simulink model "simulation_version2021b"  (R2021b)
settings: Solver=ode113  StartTime=0.0  StopTime=9  FixedStep=0.001  RelTol=1e-2
values from neighbouring files (symbols this model uses):
  b0 = 0.1    [Parameters.m]
  beta01 = 3000    [Parameters.m]
  beta02 = 100    [Parameters.m]
  beta03 = 0.01    [Parameters.m]
  d = 0.707    [Parameters.m]
  J = 8e-6    (= 8e-06)    [Parameters.m]
  k = 0.2    [Parameters.m]
  L = 0.00525    [Parameters.m]
  lambda_r = 0.0499006    [Parameters.m]
  P = 6    [Parameters.m]
  R = 7.5    [Parameters.m]
libraries: simulink x1
settings Model: Creator=49266  LastModifiedBy=49266
settings SolverCC: ZeroCrossAlgorithm=Adaptive
settings DebuggingCC: MaskedZcDiagnostic=none  IgnoredZcDiagnostic=none

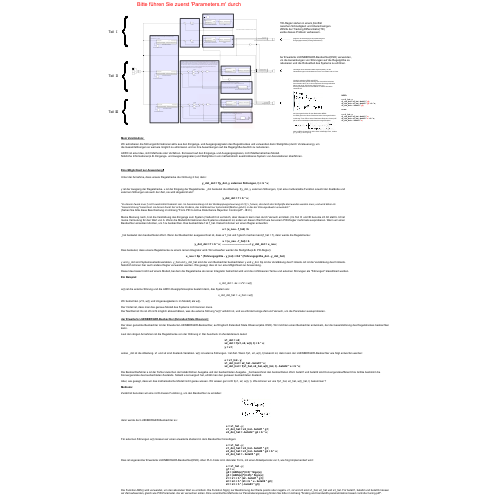
[thumbnail: Simulink's stored preview of the top-level diagram]
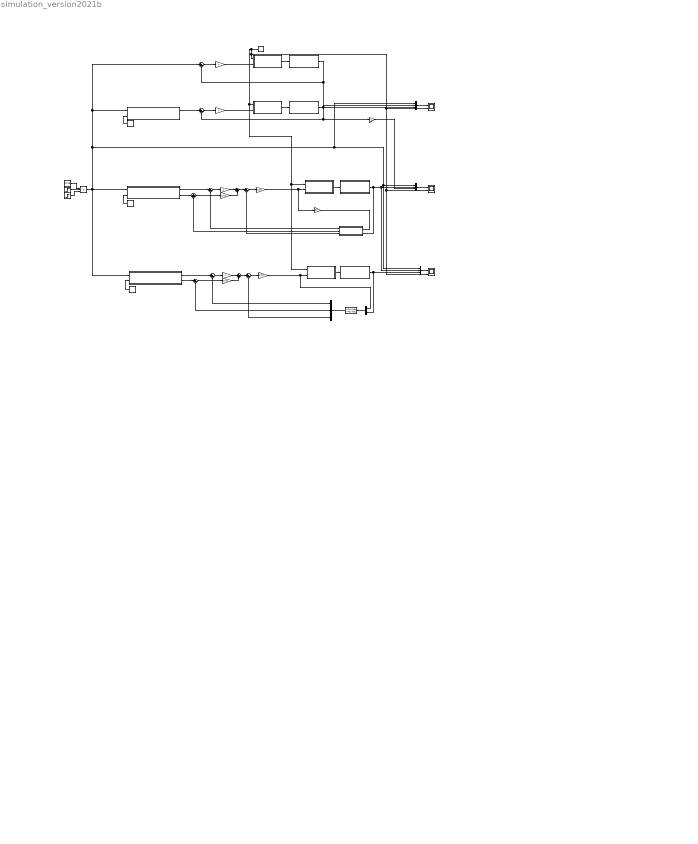
== system simulation_version2021b ==
  note: NESO:
      |
      | e = x1_hat - y;
      | x1_dot_hat = x2_hat - beta01 * g1 ;
      | x2_dot_hat = x3_hat - beta02 * g2 + b * u;
      | x3_dot_hat = - beta03 * g3 ;
  note: der Erweiterte LUENBERGER-Beobachter (Extended State Observer):
      |
      | Der oben genannte Beobachter ist der Erweiterte LUENBERGER-Beobachter, auf Englisch Extended State Observer(abk. ESO). Wir möchten einen Beobachter entwickeln, der die Gesamtstörung des Regelstreckes beobachten kann.
      |
      | Laut den obigen Annahmen ist die Regelstrecke von der Ordnung 2. Der Ausdruck im Zustandsraum lautet:
      |
      | x1_dot = x2;
      | x2_dot = f(x1, x2, w(t), t) + b * u;
      | y = x1;
      |
      | wobei _dot ist die Ableitung. x1 und x2 sind Zustand-Variablen. w(t) ist externe Störungen. t ist Zeit. Wenn f(x1, x2, w(t), t) bekannt ist, dann kann der LUENBERGER-Beobachter wie folgt entworfen werden:
      |
      | e = x1_hat - y;
      | x1_dot_hat = x2_hat - beta01 * e;
      | x2_dot_hat = f(x1_hat, x2_hat, w(t)_hat, t) - beta02 * e + b *u;
      |
      | Die Beobachterfehler e ist der Fehler zwischen der tatsächlichen Ausgabe und der beobachteten Ausgabe. _hat bezeichnet den beobachteten Wert. beta01 und beta02 sind Konvergenzkoeffizient.Ihre Größe bestimmt die Konvergenzrate des beobachteten Zustands. Sobald e konvergiert hat, erhält man den genauen beobachteten Zustand.
      |
      | Aber, wie gesagt, dass wir das mathematische Modell nicht genau wissen. Wir wissen gar nicht f(x1, x2, w(t), t). Wie können wir uns f(x1_hat, x2_hat, w(t)_hat, t) bekommen？
      |
      | Methode:
      |
      | Zunächst benutzen wir eine nicht-lineare Funktion g, um den Beobachter zu erstellen:
      |
      | dann werde der LUENBERGER-Beobachter so:
      |
      | e = x1_hat - y;
      | x1_dot_hat = x2_hat - beta01 * g1;
      | x2_dot_hat = -beta02 * g2 + b * u;
      |
      | Für externen Störungen w(t) müssen wir einen erweiterte Zustand in dem Beobachter hinzufügen:
      |
      | e = x1_hat - y;
      | x1_dot_hat = x2_hat - beta01 * g1;
      | x2_dot_hat = x3_hat - beta02 * g2 + b * u;
      | x3_dot_hat = - beta03 * g3;
      |
      | Dies ist sogenannter Erweiterte LUENBERGER-Beobachter(ESO). Aber PLC-Code ist in diskreter Form, mit einer Abtastperiode von h, wie folgt implementiert wird:
      |
      | e = x1_hat - y;
      | g1 = e;
      | g2 = (ABS(e))^(0.5) * Sign(e);
      | g3 = (ABS(e))^(0.25) * Sign(e);
      | z1 = z1 + h * (z2 - beta01 * g1);
      | z2 = z2 + h * (z3 + b * u - beta02 * g2);
      | z3 = z3 + h * (- beta03 * g3);
      |
      | Die Funktion ABS() wird verwendet, um den absoluten Wert zu ermitteln. Die Funktion Sign() zur Bestimmung der Werte positiv oder negativ. z1, z2 und z3 sind x1_hat, x2_hat und x3_hat. Für beta01, beta02 und beta03 müssen wir Zeit aufwenden, gleich wie PID-Parameter. die wir versuchen sollen. Eine vereinfachte Methode zur Parameteranpassung finden Sie bitte im Anhang "Scaling and bandwidth-parametrization based controller tuning.pdf".
  note: der Erweiterte LUENBERGER-Beobachter(ESO) verwenden, um die Auswirkungen von Störungen auf die Regelgröße zu reduzieren und die Robustheit des Systems zu erhöhen.
  note: PID-Regler stehen in einem Konflikt zwischen Schnelligkeit und Überschwingen.
      | Mithilfe der Tracking Differentiator(TD) werde dieses Problem verbessern.
  note: Regelstrecke
  note: Regelstrecke
  note: Regelstrecke
  note: Regelstrecke
  note: Bitte führen Sie zuerst 'Parameters.m' durch
  note: Eine Möglichkeit zur Anwendung：
      |
      | Unter der Annahme, dass unsere Regelstrecke die Ordnung 2 hat, dann:
      |
      | y_dot_dot = f(y_dot, y, externen Störungen, t) + b * u;
      |
      | y ist der Ausgang der Regelstrecke. u ist der Eingang der Regelstrecke. _dot bedeutet die Ableitung. f(y_dot, y, externen Störungen, t) ist eine multivariable Funktion sowohl der Zustände und externen Störungen als auch der Zeit, sie wird abgekürzt als f：
      |
      | y_dot_dot = f + b * u;
      |
      | "Zu diesem Zweck muss f nicht ausdrücklich bekannt sein. Im Zusammenhang mit der Rückkopplungssteuerung ist F(t) = f etwas, das durch das Stellgröße überwunden werden muss, und wird daher als "Gesamtstörung" bezeichnet. An diesem Punkt hat sich das Problem, das traditionell zur Systemidentifikation gehört, in das der Störungsabwehr verwandelt."
      | (Sehen Sie bitte diese Beschreibung im Anhang "From PID to Active Disturbance Rejection Control.pdf" - Ⅲ.D.)
      |
      | Meine Meinung nach, b ist die Verstärkung des Eingangs zum System.(Vielleicht ist es falsch, aber dieses b kann man durch Versuch ermitteln.) Im Teil Ⅱ und Ⅲ benutze ich b0 statt b. b0 ist meine Vermutung für den Wert von b. Wenn die Modellinformationen des Systems unbekannt ist, sollen wir diesen Wert b0 wie bei einem PID-Regler mehrmals ausprobieren. Wenn wir einen Beobachter einsetzen könnten, um f zu beobachten. Das beobachtete f ist f_hat. Danach können wir einen Regler entwerfen:
      |
      | u = (u_neu - f_hat) / b
      |
      | _hat bedeutet den beobachteten Wert. Wenn der Beobachter ausgezeichnet ist, dass er f_hat und f gleich machen kann(f_hat = f), dann werde die Regelstrecke:
      |
      | u = (u_neu - f_hat) / b
      | y_dot_dot = f + b * u; -------------------------------> y_dot_dot = u_neu;
      |
      | Dies bedeutet, dass unsere Regelstrecke zu einem reinen Integrator wird. Wir entwerfen weriter die Stellgröße(z.B. PD-Regler):
      |
      | u_neu = Kp * (Führungsgröße - y_hat) + Kd * (Führungsgröße_dot - y_dot_hat)
      |
      | y und y_dot sind Systemzustandsvariablen. y_hat und y_dot_hat sind die vom Beobachter beobachteten y und y_dot. Kp ist die Verstärkung des P-Glieds. kd ist die Verstärkung des D-Glieds. Natürlich können hier auch andere Regler verwendet werden. Wie gesagt, dies ist nur eine Möglichkeit zur Anwendung.
      |
      | Diese Idee basiert nicht auf einem Modell, bei dem die Regelstrecke als reiner Integrator betrachtet wird und die nichtlinearen Terme und externen Störungen als "Störungen" klassifiziert werden.
      |
      | Ein Beispiel:
      |
      | x_dot_dot = -kx + x^2 + w(t)
      |
      | w(t) ist die externe Störung und die ADRC-Designphilosophie besteht darin, das System als:
      |
      | x_dot_dot_hat = -x_hat + w(t)
      |
      | Wir betrachten (x^2, w(t) und Ungenauigkeiten k im Modell) als w(t).
      |
      | Der Vorteil ist, dass man das genaue Modell des Systems nicht kennen muss.
      | Der Nachteil ist: Es ist oft nicht möglich abzuschätzen, was die externe Störung "w(t)" wirklich ist, und es erfordert einige Zeit und Versuch, um die Parameter auszuprobieren.
  note: Mein Verständnis:
      |
      | Wir extrahieren die Störungsinformationen aktiv aus den Eingangs- und Ausgangssignalen des Regelstreckes und verwenden dann Stellgröße (durch Vorsteuerung), um die Gesamtstörungen so weit wie möglich zu eliminieren und so ihre Auswirkungen auf die Regelgröße deutlich zu reduzieren.
      |
      | ADRC ist eine Idee, nicht Methode oder Verfahren. Es basiert auf den Eingangs- und Ausgangssignalen, nicht Mathematisches Modell.
      | Nützliche Informationen(z.B. Eingangs- und Ausgangssignalen) und Stellgröße in ein mathematisch ausdrückbares System von Assoziationen überführen.
  note: Teil Ⅰ
  note: nomaler PID-Regler mit Feedback-Kreis
  note: Linear Extended State Observer (LESO)
      | ist der Erweiterte Lineare LUENBERGER-Beobachter
  note: Nicht-linear Extended State Observer (NESO)
      | ist der Erweiterte Nicht-lineare LUENBERGER-Beobachter
  note: Tracking Differentiator(TD) is a Transient Profile Generator.
      | Um den Konflikt zwischen Schnelligkeit und Überschwingen
      | bei PID-Reglern zu lösen.
  note: Nonlinear Feedback Combination is a Nonlinear Weighted Sum(eigentlich ein PD-Regler).
      | Der ESO ist eigentlich eine Erweiterung des Luenberger Observers mit einer erweiterten Zustand.
      | Dieser erweiterter Zustand wird verwendet, um (den unbekannten Term + externen Störungen +
      | den nicht-linearen Term) zu ermitteln. Dies wird in Abschnitt III.D. der Dissertation beschrieben.
      |
      | Wenn der Extended State Observer (ESO) die Unbekannte(z3) sehr genau ermitteln kann,
      | dann wird die Regelstrecke zu einem reinen Integrator.
  note: Teil Ⅱ
  note: Teil Ⅲ
  note: Vergleich: die Auswirkungen der Anwendung des Übergangsprozesses(Tracking Differentiator)
  note: Hinzufügen eines Extended State Observer(ESO), um die Gesamtstörungen und unbekannten Terme zu ermitteln und zu lösen.
  note: Vergleich zwischen LESO und NESO.
      | Sie haben die fast gleiche Wirkung. Der Unterschied zwischen ihnen besteht darin, ob sie eine nichtlineare Konvergenzfunktion haben oder nicht. Wir können viele Formen von Konvergenzfunktionen für ESO wählen. In dieser Simulation verwende ich
      |
      | als Konvergenzfunktion für den Beobachter NESO.
      | Im LESO gibt es bei dieser Simulation keine Konvergenzfunktion.
      |
      | im Anhang "From PID to Active Disturbance Rejection Control.pdf" gibt es eine vollständige nichtlineare Konvergenzfunktion.
      |
      | Aber in NESO verwende ich nicht diese vollständige Form, sondern g1, g2 und g3. Es ist genug.
  note: LESO:
      |
      | e = x1_hat - y;
      | x1_dot_hat = x2_hat - beta01 * e ;
      | x2_dot_hat = x3_hat - beta02 * e + b * u;
      | x3_dot_hat = - beta03 * e ;
  1/b0 : Gain  Gain=1/b0
  1/b0_1 : Gain  Gain=1/b0
  Aktor(Fadenzugmotor)3 : Subsystem
  Aktor(Servoverstäker+Fadenzugmotor) : Subsystem
  Aktor(Servoverstäker+Fadenzugmotor)1 : Subsystem
  Aktor(Servoverstäker+Fadenzugmotor)2 : Subsystem
  D-Glied : Gain  Gain=0.01
  D-Glied1 : Gain  Gain=0.01
  Demux : Demux  Outputs=3
  Externe Störungen(Einheit: Nm) Motor Rated Torque Mn = 0.38N : simulink/Sources/Band-Limited White Noise  Cov=[0.002]  Ts=0.1  seed=[23341]
  Faden : Subsystem
  Faden1 : Subsystem
  Faden2 : Subsystem
  Faden3 : Subsystem
  Führungsgröße : Product  Inputs=3
  Konvergenzgeschwindigkeit : Constant  Value=2000
  Konvergenzgeschwindigkeit1 : Constant  Value=2000
  Konvergenzgeschwindigkeit2 : Constant  Value=2000
  Linear Extended State Observer (LESO) : StateSpace  A=[-beta01 1 0;-beta02 0 1;-beta03 0 0]  B=[0 beta01;b0 beta02;0 beta03]  C=[1 0 0;0 1 0;0 0 1]  D=[0 0;0 0;0 0]  InitialCondition=0
  Mux : Mux  Inputs=2
  Mux1 : Mux  Inputs=3
  Mux2 : Mux  Inputs=3
  Mux3 : Mux  Inputs=3
  Nicht-linear Extended State Observer (NESO) : Subsystem
  P-Glied{,1..3} (4 alike) : Gain
  Pulse Generator : DiscretePulseGenerator  PulseType=Time based  Amplitude=10  Period=5  PulseWidth=50
  Scope : Scope  NumInputPorts=2
  Scope1 : Scope  NumInputPorts=2
  Scope4 : Scope  NumInputPorts=2
  Step1 : Step  Time=5  Before=1  After=0.5  SampleTime=0
  Step2 : Step  Time=10  Before=1  After=1.5  SampleTime=0
  Sum{,1..3,5,7,9..10} (8 alike) : Sum  Inputs=|+-
  Sum4 : Sum  Inputs=|++
  Sum6 : Sum  Inputs=|++
  Tracking Differentiator(TD) : Subsystem
  Tracking Differentiator(TD)1 : Subsystem
  Tracking Differentiator(TD)2 : Subsystem
  "Um Signal zu umbenennen " : Gain
  b0 : Gain  Gain=b0
  wires:
  Externe Störungen(Einheit: Nm) Motor Rated Torque Mn = 0.38N/1 -> Aktor(Servoverstäker+Fadenzugmotor)1/1(externen Störungen), Aktor(Fadenzugmotor)3/1(externen Störungen), Aktor(Servoverstäker+Fadenzugmotor)2/1(externen Störungen), Scope4/2, Scope1/2, Scope/2, Aktor(Servoverstäker+Fadenzugmotor)/1(externen Störungen)  "Externe Störungen(Einheit: N.m) Motor Rated Torque Mn = 0.38Nm"
  Faden3/1(Fadenzugspannung) -> Mux/2, Mux3/3  "Regelgröße mit LESO"
  Aktor(Fadenzugmotor)3/1(Position) -> Faden3/1(Verdrängung)
  Linear Extended State Observer (LESO)/1 -> Demux/1
  Mux/1 -> Linear Extended State Observer (LESO)/1
  Führungsgröße/1 -> Sum/1, Tracking Differentiator(TD)2/1(Führungsgröße), Mux1/1, Mux3/1, Mux2/1, Tracking Differentiator(TD)/1(Führungsgröße), Tracking Differentiator(TD)1/1(Führungsgröße)  "Führungsgröße"
  P-Glied/1 -> Aktor(Servoverstäker+Fadenzugmotor)/2(Fadenzugspannung)
  Tracking Differentiator(TD)2/1(Übergangskurve) -> Sum1/1
  Step2/1 -> Führungsgröße/3
  Faden2/1(Fadenzugspannung) -> Sum1/2, "Um Signal zu umbenennen "/1, Mux1/3  "mit Tracking Differentiator"
  Sum/1 -> P-Glied/1
  Konvergenzgeschwindigkeit/1 -> Tracking Differentiator(TD)2/2(Konvergenzgeschwindigkeit)
  Pulse Generator/1 -> Führungsgröße/1
  Sum1/1 -> P-Glied1/1
  Step1/1 -> Führungsgröße/2
  P-Glied1/1 -> Aktor(Servoverstäker+Fadenzugmotor)2/2(Fadenzugspannung)
  Faden/1(Fadenzugspannung) -> Mux1/2, Sum/2  "ohne Tracking Differentiator"
  Aktor(Servoverstäker+Fadenzugmotor)/1(Position) -> Faden/1(Verdrängung)
  Aktor(Servoverstäker+Fadenzugmotor)2/1(Position) -> Faden2/1(Verdrängung)
  Aktor(Servoverstäker+Fadenzugmotor)1/1(Position) -> Faden1/1(Verdrängung)
  Faden1/1(Fadenzugspannung) -> Mux3/2, Mux2/2, Nicht-linear Extended State Observer (NESO)/2(y)  "Regelgröße mit ESO"
  Tracking Differentiator(TD)/1(Übergangskurve) -> Sum2/1
  Sum2/1 -> P-Glied3/1
  Konvergenzgeschwindigkeit1/1 -> Tracking Differentiator(TD)/2(Konvergenzgeschwindigkeit)
  Nicht-linear Extended State Observer (NESO)/1(Z1) -> Sum2/2  "x1_hat"
  P-Glied3/1 -> Sum4/1
  Sum4/1 -> Sum9/1
  Tracking Differentiator(TD)/2(Ableitungen der Übergangskurven) -> Sum10/1
  Nicht-linear Extended State Observer (NESO)/2(Z2) -> Sum10/2  "x2_hat"
  Sum10/1 -> D-Glied/1
  Nicht-linear Extended State Observer (NESO)/3(Z3) -> Sum9/2  "x3_hat：total disturbance (Beobachtete Gesamtstörung)"
  Sum9/1 -> 1/b0/1
  1/b0/1 -> b0/1, Aktor(Servoverstäker+Fadenzugmotor)1/2(Fadenzugspannung)
  b0/1 -> Nicht-linear Extended State Observer (NESO)/1(u)
  Demux/3 -> Sum7/2  "x3_hat：total disturbance (Beobachtete Gesamtstörung)"
  Demux/1 -> Sum5/2  "x1_hat"
  Demux/2 -> Sum3/2  "x2_hat"
  D-Glied1/1 -> Sum6/2
  Sum7/1 -> 1/b0_1/1
  1/b0_1/1 -> Mux/1, Aktor(Fadenzugmotor)3/2(Fadenzugspannung)
  Sum3/1 -> D-Glied1/1
  Sum6/1 -> Sum7/1
  P-Glied2/1 -> Sum6/1
  Sum5/1 -> P-Glied2/1
  Konvergenzgeschwindigkeit2/1 -> Tracking Differentiator(TD)1/2(Konvergenzgeschwindigkeit)
  Tracking Differentiator(TD)1/1(Übergangskurve) -> Sum5/1
  Tracking Differentiator(TD)1/2(Ableitungen der Übergangskurven) -> Sum3/1
  "Um Signal zu umbenennen "/1 -> Mux2/3  "Regelgröße ohne ESO"
  Mux1/1 -> Scope/1
  Mux2/1 -> Scope4/1
  Mux3/1 -> Scope1/1
  D-Glied/1 -> Sum4/2

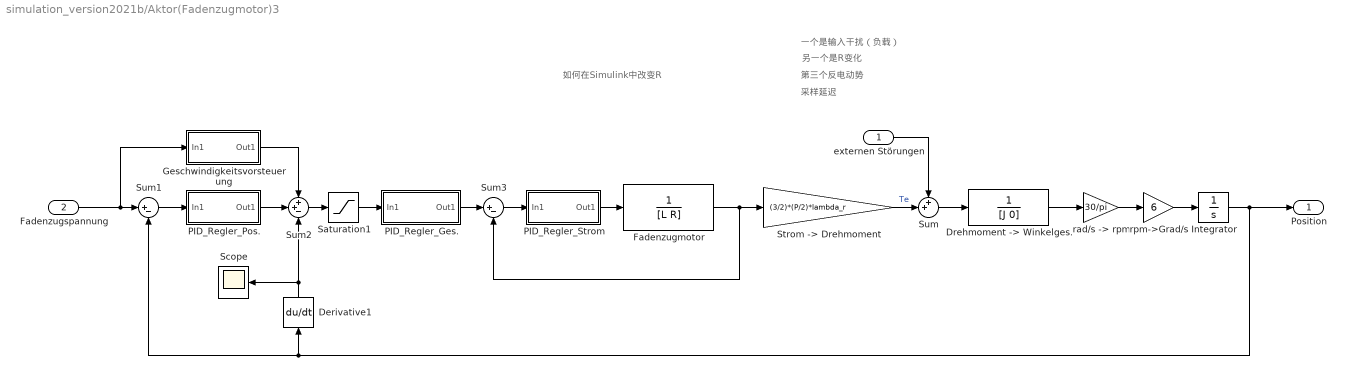
== system simulation_version2021b/Aktor(Fadenzugmotor)3 ==
  note: 采样延迟
  note: 第三个反电动势
  note: 另一个是R变化
  note: 一个是输入干扰（负载）
  note: 如何在Simulink中改变R
  externen Störungen : Inport
  Fadenzugspannung : Inport  Port=2
  Derivative1 : Derivative
  "Drehmoment -> Winkelges." : TransferFcn  Denominator=[J 0]
  Fadenzugmotor : TransferFcn  Denominator=[L R]
  Geschwindigkeitsvorsteuerung : Subsystem
  Integrator : Integrator
  PID_Regler_Ges. : Subsystem
  PID_Regler_Pos. : Subsystem
  PID_Regler_Strom : Subsystem
  Saturation1 : Saturate  UpperLimit=9500  LowerLimit=-9500
  Scope : Scope
  "Strom -> Drehmoment" : Gain  Gain=(3/2)*(P/2)*lambda_r
  Sum : Sum  Inputs=++|
  Sum1 : Sum  Inputs=|+-
  Sum2 : Sum  Inputs=++-
  Sum3 : Sum  Inputs=|+-
  "rad/s -> rpm" : Gain  Gain=30/pi
  rpm->Grad/s : Gain  Gain=6
  Position : Outport
  wires:
  "Drehmoment -> Winkelges."/1 -> "rad/s -> rpm"/1
  Derivative1/1 -> Sum2/3, Scope/1
  Fadenzugspannung/1 -> Geschwindigkeitsvorsteuerung/1(In1), Sum1/1
  rpm->Grad/s/1 -> Integrator/1
  "rad/s -> rpm"/1 -> rpm->Grad/s/1
  Integrator/1 -> Position/1, Derivative1/1, Sum1/2
  Fadenzugmotor/1 -> "Strom -> Drehmoment"/1, Sum3/2
  "Strom -> Drehmoment"/1 -> Sum/2  "Te"
  Sum/1 -> "Drehmoment -> Winkelges."/1
  externen Störungen/1 -> Sum/1
  Sum2/1 -> Saturation1/1
  Saturation1/1 -> PID_Regler_Ges./1(In1)
  PID_Regler_Ges./1(Out1) -> Sum3/1
  Sum1/1 -> PID_Regler_Pos./1(In1)
  PID_Regler_Pos./1(Out1) -> Sum2/2
  Geschwindigkeitsvorsteuerung/1(Out1) -> Sum2/1
  Sum3/1 -> PID_Regler_Strom/1(In1)
  PID_Regler_Strom/1(Out1) -> Fadenzugmotor/1

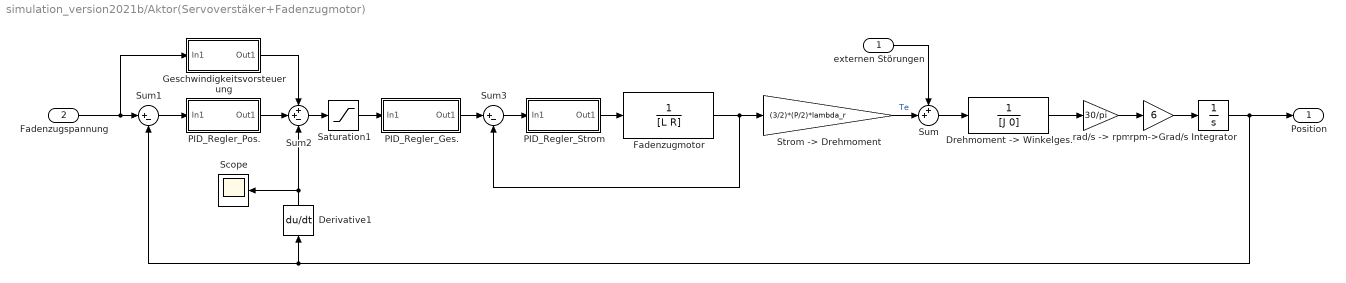
== system simulation_version2021b/Aktor(Servoverstäker+Fadenzugmotor) ==
  externen Störungen : Inport
  Fadenzugspannung : Inport  Port=2
  Derivative1 : Derivative
  "Drehmoment -> Winkelges." : TransferFcn  Denominator=[J 0]
  Fadenzugmotor : TransferFcn  Denominator=[L R]
  Geschwindigkeitsvorsteuerung : Subsystem
  Integrator : Integrator
  PID_Regler_Ges. : Subsystem
  PID_Regler_Pos. : Subsystem
  PID_Regler_Strom : Subsystem
  Saturation1 : Saturate  UpperLimit=9500  LowerLimit=-9500
  Scope : Scope
  "Strom -> Drehmoment" : Gain  Gain=(3/2)*(P/2)*lambda_r
  Sum : Sum  Inputs=++|
  Sum1 : Sum  Inputs=|+-
  Sum2 : Sum  Inputs=++-
  Sum3 : Sum  Inputs=|+-
  "rad/s -> rpm" : Gain  Gain=30/pi
  rpm->Grad/s : Gain  Gain=6
  Position : Outport
  wires:
  "Drehmoment -> Winkelges."/1 -> "rad/s -> rpm"/1
  Derivative1/1 -> Sum2/3, Scope/1
  Fadenzugspannung/1 -> Geschwindigkeitsvorsteuerung/1(In1), Sum1/1
  rpm->Grad/s/1 -> Integrator/1
  "rad/s -> rpm"/1 -> rpm->Grad/s/1
  Integrator/1 -> Position/1, Derivative1/1, Sum1/2
  Fadenzugmotor/1 -> "Strom -> Drehmoment"/1, Sum3/2
  "Strom -> Drehmoment"/1 -> Sum/2  "Te"
  Sum/1 -> "Drehmoment -> Winkelges."/1
  externen Störungen/1 -> Sum/1
  Sum2/1 -> Saturation1/1
  Saturation1/1 -> PID_Regler_Ges./1(In1)
  PID_Regler_Ges./1(Out1) -> Sum3/1
  Sum1/1 -> PID_Regler_Pos./1(In1)
  PID_Regler_Pos./1(Out1) -> Sum2/2
  Geschwindigkeitsvorsteuerung/1(Out1) -> Sum2/1
  Sum3/1 -> PID_Regler_Strom/1(In1)
  PID_Regler_Strom/1(Out1) -> Fadenzugmotor/1

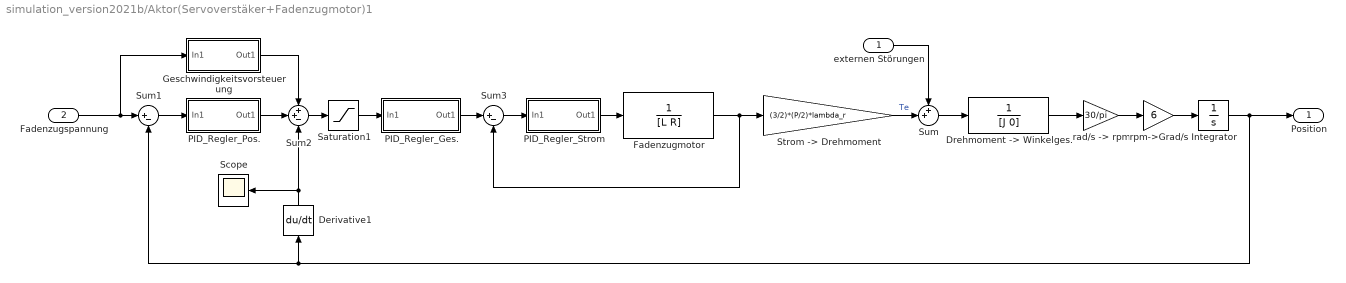
== system simulation_version2021b/Aktor(Servoverstäker+Fadenzugmotor)1 ==
  externen Störungen : Inport
  Fadenzugspannung : Inport  Port=2
  Derivative1 : Derivative
  "Drehmoment -> Winkelges." : TransferFcn  Denominator=[J 0]
  Fadenzugmotor : TransferFcn  Denominator=[L R]
  Geschwindigkeitsvorsteuerung : Subsystem
  Integrator : Integrator
  PID_Regler_Ges. : Subsystem
  PID_Regler_Pos. : Subsystem
  PID_Regler_Strom : Subsystem
  Saturation1 : Saturate  UpperLimit=9500  LowerLimit=-9500
  Scope : Scope
  "Strom -> Drehmoment" : Gain  Gain=(3/2)*(P/2)*lambda_r
  Sum : Sum  Inputs=++|
  Sum1 : Sum  Inputs=|+-
  Sum2 : Sum  Inputs=++-
  Sum3 : Sum  Inputs=|+-
  "rad/s -> rpm" : Gain  Gain=30/pi
  rpm->Grad/s : Gain  Gain=6
  Position : Outport
  wires:
  "Drehmoment -> Winkelges."/1 -> "rad/s -> rpm"/1
  Derivative1/1 -> Sum2/3, Scope/1
  Fadenzugspannung/1 -> Geschwindigkeitsvorsteuerung/1(In1), Sum1/1
  rpm->Grad/s/1 -> Integrator/1
  "rad/s -> rpm"/1 -> rpm->Grad/s/1
  Integrator/1 -> Position/1, Derivative1/1, Sum1/2
  Fadenzugmotor/1 -> "Strom -> Drehmoment"/1, Sum3/2
  "Strom -> Drehmoment"/1 -> Sum/2  "Te"
  Sum/1 -> "Drehmoment -> Winkelges."/1
  externen Störungen/1 -> Sum/1
  Sum2/1 -> Saturation1/1
  Saturation1/1 -> PID_Regler_Ges./1(In1)
  PID_Regler_Ges./1(Out1) -> Sum3/1
  Sum1/1 -> PID_Regler_Pos./1(In1)
  PID_Regler_Pos./1(Out1) -> Sum2/2
  Geschwindigkeitsvorsteuerung/1(Out1) -> Sum2/1
  Sum3/1 -> PID_Regler_Strom/1(In1)
  PID_Regler_Strom/1(Out1) -> Fadenzugmotor/1

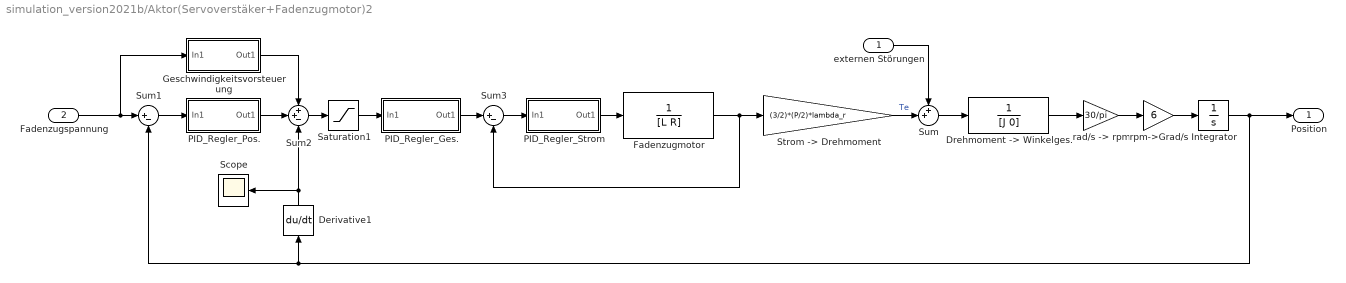
== system simulation_version2021b/Aktor(Servoverstäker+Fadenzugmotor)2 ==
  externen Störungen : Inport
  Fadenzugspannung : Inport  Port=2
  Derivative1 : Derivative
  "Drehmoment -> Winkelges." : TransferFcn  Denominator=[J 0]
  Fadenzugmotor : TransferFcn  Denominator=[L R]
  Geschwindigkeitsvorsteuerung : Subsystem
  Integrator : Integrator
  PID_Regler_Ges. : Subsystem
  PID_Regler_Pos. : Subsystem
  PID_Regler_Strom : Subsystem
  Saturation1 : Saturate  UpperLimit=9500  LowerLimit=-9500
  Scope : Scope
  "Strom -> Drehmoment" : Gain  Gain=(3/2)*(P/2)*lambda_r
  Sum : Sum  Inputs=++|
  Sum1 : Sum  Inputs=|+-
  Sum2 : Sum  Inputs=++-
  Sum3 : Sum  Inputs=|+-
  "rad/s -> rpm" : Gain  Gain=30/pi
  rpm->Grad/s : Gain  Gain=6
  Position : Outport
  wires:
  "Drehmoment -> Winkelges."/1 -> "rad/s -> rpm"/1
  Derivative1/1 -> Sum2/3, Scope/1
  Fadenzugspannung/1 -> Geschwindigkeitsvorsteuerung/1(In1), Sum1/1
  rpm->Grad/s/1 -> Integrator/1
  "rad/s -> rpm"/1 -> rpm->Grad/s/1
  Integrator/1 -> Position/1, Derivative1/1, Sum1/2
  Fadenzugmotor/1 -> "Strom -> Drehmoment"/1, Sum3/2
  "Strom -> Drehmoment"/1 -> Sum/2  "Te"
  Sum/1 -> "Drehmoment -> Winkelges."/1
  externen Störungen/1 -> Sum/1
  Sum2/1 -> Saturation1/1
  Saturation1/1 -> PID_Regler_Ges./1(In1)
  PID_Regler_Ges./1(Out1) -> Sum3/1
  Sum1/1 -> PID_Regler_Pos./1(In1)
  PID_Regler_Pos./1(Out1) -> Sum2/2
  Geschwindigkeitsvorsteuerung/1(Out1) -> Sum2/1
  Sum3/1 -> PID_Regler_Strom/1(In1)
  PID_Regler_Strom/1(Out1) -> Fadenzugmotor/1

== system simulation_version2021b/Faden ==
  Verdrängung : Inport
  Transfer Fcn : TransferFcn  Numerator=[400]  Denominator=[d k]
  Fadenzugspannung : Outport
  wires:
  Verdrängung/1 -> Transfer Fcn/1
  Transfer Fcn/1 -> Fadenzugspannung/1

== system simulation_version2021b/Faden1 ==
  Verdrängung : Inport
  Transfer Fcn : TransferFcn  Numerator=[400]  Denominator=[d k]
  Fadenzugspannung : Outport
  wires:
  Verdrängung/1 -> Transfer Fcn/1
  Transfer Fcn/1 -> Fadenzugspannung/1

== system simulation_version2021b/Faden2 ==
  Verdrängung : Inport
  Transfer Fcn : TransferFcn  Numerator=[400]  Denominator=[d k]
  Fadenzugspannung : Outport
  wires:
  Transfer Fcn/1 -> Fadenzugspannung/1
  Verdrängung/1 -> Transfer Fcn/1

== system simulation_version2021b/Faden3 ==
  Verdrängung : Inport
  Transfer Fcn : TransferFcn  Numerator=[400]  Denominator=[d k]
  Fadenzugspannung : Outport
  wires:
  Transfer Fcn/1 -> Fadenzugspannung/1
  Verdrängung/1 -> Transfer Fcn/1

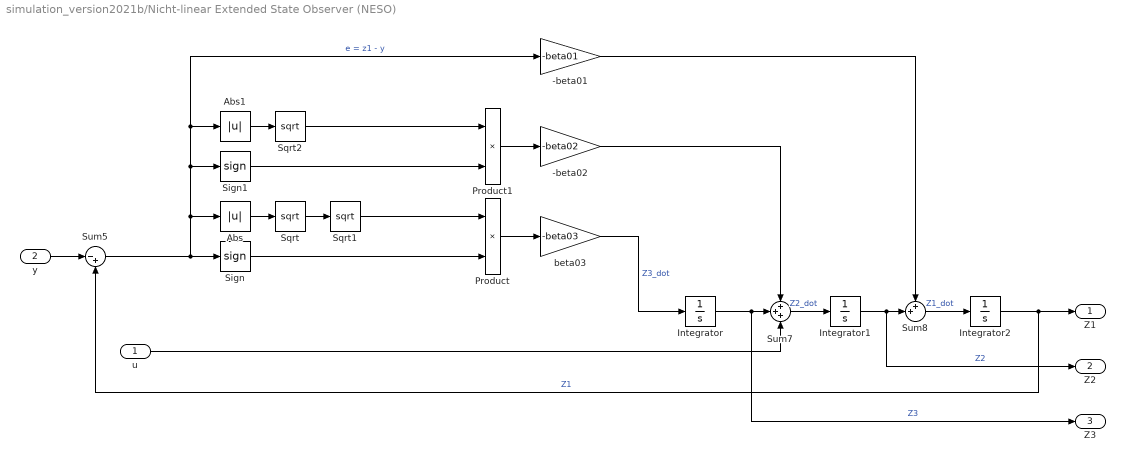
== system simulation_version2021b/Nicht-linear Extended State Observer (NESO) ==
  u : Inport
  y : Inport  Port=2
  -beta01 : Gain  Gain=-beta01
  -beta02 : Gain  Gain=-beta02
  Abs : Abs
  Abs1 : Abs
  Integrator : Integrator
  Integrator1 : Integrator
  Integrator2 : Integrator
  Product : Product
  Product1 : Product
  Sign : Signum
  Sign1 : Signum
  Sqrt : Sqrt  SaturateOnIntegerOverflow=on
  Sqrt1 : Sqrt  SaturateOnIntegerOverflow=on
  Sqrt2 : Sqrt  SaturateOnIntegerOverflow=on
  Sum5 : Sum  Inputs=|-+
  Sum7 : Sum  Inputs=+++
  Sum8 : Sum  Inputs=++|
  beta03 : Gain  Gain=-beta03
  Z1 : Outport
  Z2 : Outport  Port=2
  Z3 : Outport  Port=3
  wires:
  Abs/1 -> Sqrt/1
  Sqrt/1 -> Sqrt1/1
  beta03/1 -> Integrator/1  "Z3_dot"
  Integrator1/1 -> Sum8/2, Z2/1  "Z2"
  Sum5/1 -> Sign1/1, -beta01/1, Abs1/1, Abs/1, Sign/1  "e = z1 - y"
  Integrator2/1 -> Z1/1, Sum5/2  "Z1"
  Sign1/1 -> Product1/2
  Abs1/1 -> Sqrt2/1
  Sum8/1 -> Integrator2/1  "Z1_dot"
  Sum7/1 -> Integrator1/1  "Z2_dot"
  Product1/1 -> -beta02/1
  -beta02/1 -> Sum7/1
  Product/1 -> beta03/1
  -beta01/1 -> Sum8/1
  Sign/1 -> Product/2
  Integrator/1 -> Z3/1, Sum7/2  "Z3"
  y/1 -> Sum5/1
  Sqrt1/1 -> Product/1
  u/1 -> Sum7/3
  Sqrt2/1 -> Product1/1

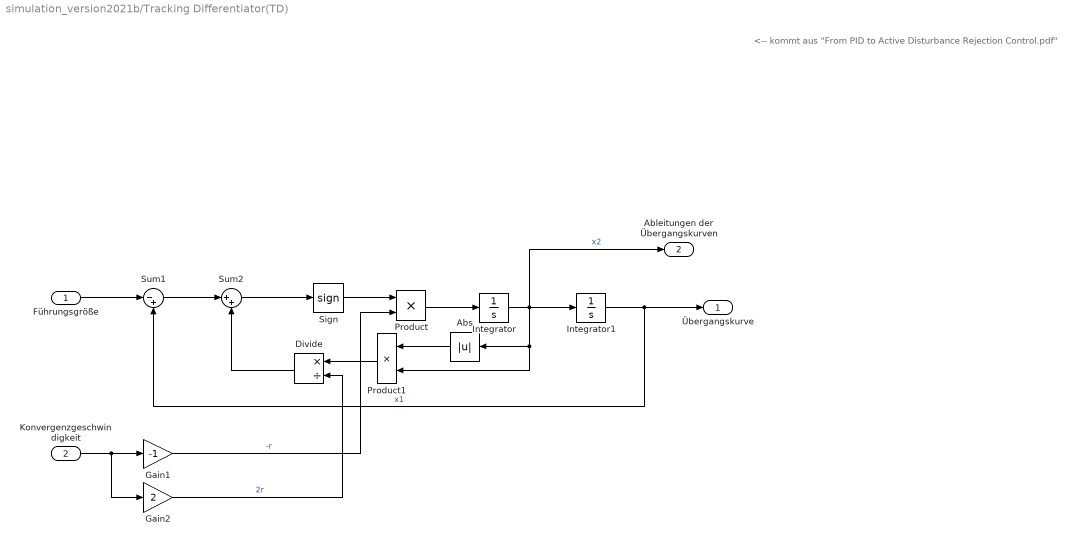
== system simulation_version2021b/Tracking Differentiator(TD) ==
  note: <-- kommt aus "From PID to Active Disturbance Rejection Control.pdf"
  Führungsgröße : Inport
  Konvergenzgeschwindigkeit : Inport  Port=2
  Abs : Abs
  Divide : Product  Inputs=*/
  Gain1 : Gain  Gain=-1
  Gain2 : Gain  Gain=2
  Integrator : Integrator
  Integrator1 : Integrator
  Product : Product
  Product1 : Product
  Sign : Signum
  Sum1 : Sum  Inputs=|-+
  Sum2 : Sum  Inputs=|++
  Übergangskurve : Outport
  Ableitungen der Übergangskurven : Outport  Port=2
  wires:
  Sum1/1 -> Sum2/1
  Product1/1 -> Divide/1
  Konvergenzgeschwindigkeit/1 -> Gain2/1, Gain1/1
  Führungsgröße/1 -> Sum1/1
  Integrator/1 -> Ableitungen der Übergangskurven/1, Integrator1/1, Product1/2, Abs/1  "x2"
  Divide/1 -> Sum2/2
  Integrator1/1 -> Übergangskurve/1, Sum1/2  "x1"
  Product/1 -> Integrator/1
  Abs/1 -> Product1/1
  Sum2/1 -> Sign/1
  Gain1/1 -> Product/2  "-r"
  Sign/1 -> Product/1
  Gain2/1 -> Divide/2  "2r"

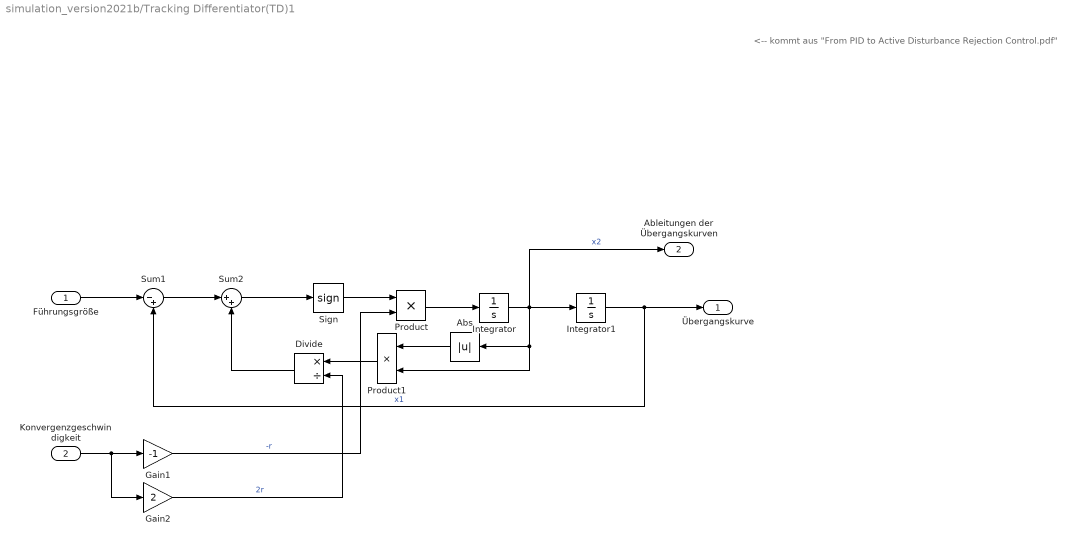
== system simulation_version2021b/Tracking Differentiator(TD)1 ==
  note: <-- kommt aus "From PID to Active Disturbance Rejection Control.pdf"
  Führungsgröße : Inport
  Konvergenzgeschwindigkeit : Inport  Port=2
  Abs : Abs
  Divide : Product  Inputs=*/
  Gain1 : Gain  Gain=-1
  Gain2 : Gain  Gain=2
  Integrator : Integrator
  Integrator1 : Integrator
  Product : Product
  Product1 : Product
  Sign : Signum
  Sum1 : Sum  Inputs=|-+
  Sum2 : Sum  Inputs=|++
  Übergangskurve : Outport
  Ableitungen der Übergangskurven : Outport  Port=2
  wires:
  Sum1/1 -> Sum2/1
  Product1/1 -> Divide/1
  Konvergenzgeschwindigkeit/1 -> Gain2/1, Gain1/1
  Führungsgröße/1 -> Sum1/1
  Integrator/1 -> Ableitungen der Übergangskurven/1, Integrator1/1, Product1/2, Abs/1  "x2"
  Divide/1 -> Sum2/2
  Integrator1/1 -> Übergangskurve/1, Sum1/2  "x1"
  Product/1 -> Integrator/1
  Abs/1 -> Product1/1
  Sum2/1 -> Sign/1
  Gain1/1 -> Product/2  "-r"
  Sign/1 -> Product/1
  Gain2/1 -> Divide/2  "2r"

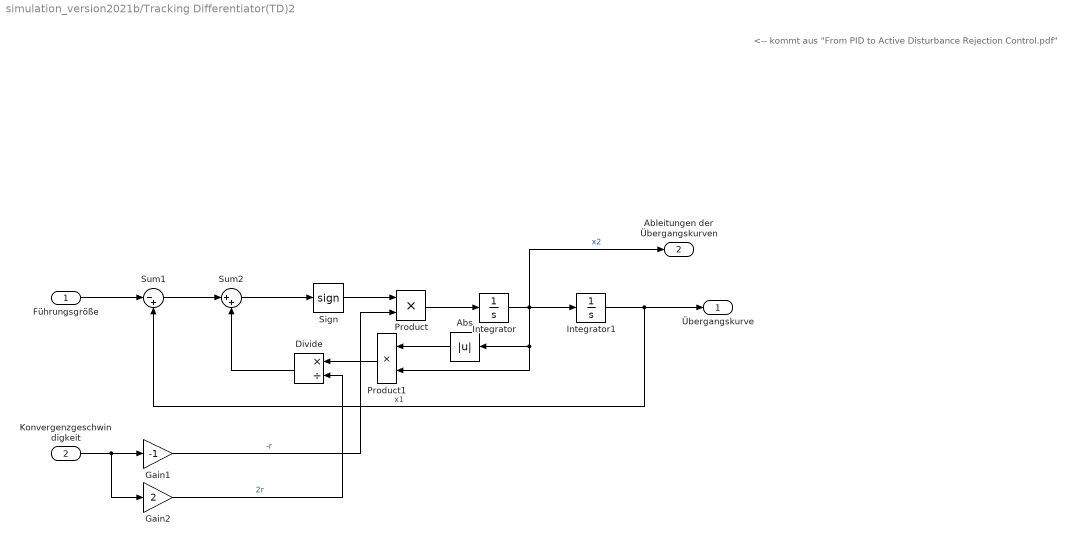
== system simulation_version2021b/Tracking Differentiator(TD)2 ==
  note: <-- kommt aus "From PID to Active Disturbance Rejection Control.pdf"
  Führungsgröße : Inport
  Konvergenzgeschwindigkeit : Inport  Port=2
  Abs : Abs
  Divide : Product  Inputs=*/
  Gain1 : Gain  Gain=-1
  Gain2 : Gain  Gain=2
  Integrator : Integrator
  Integrator1 : Integrator
  Product : Product
  Product1 : Product
  Sign : Signum
  Sum1 : Sum  Inputs=|-+
  Sum2 : Sum  Inputs=|++
  Übergangskurve : Outport
  Ableitungen der Übergangskurven : Outport  Port=2
  wires:
  Gain2/1 -> Divide/2  "2r"
  Sign/1 -> Product/1
  Gain1/1 -> Product/2  "-r"
  Sum2/1 -> Sign/1
  Abs/1 -> Product1/1
  Product/1 -> Integrator/1
  Integrator1/1 -> Sum1/2, Übergangskurve/1  "x1"
  Divide/1 -> Sum2/2
  Integrator/1 -> Abs/1, Product1/2, Integrator1/1, Ableitungen der Übergangskurven/1  "x2"
  Führungsgröße/1 -> Sum1/1
  Konvergenzgeschwindigkeit/1 -> Gain1/1, Gain2/1
  Product1/1 -> Divide/1
  Sum1/1 -> Sum2/1

== system simulation_version2021b/Aktor(Fadenzugmotor)3/Geschwindigkeitsvorsteuerung ==
  In1 : Inport
  Derivative : Derivative
  Gain : Gain
  Out1 : Outport
  wires:
  Derivative/1 -> Gain/1
  In1/1 -> Derivative/1
  Gain/1 -> Out1/1

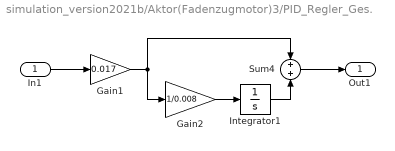
== system simulation_version2021b/Aktor(Fadenzugmotor)3/PID_Regler_Ges. ==
  In1 : Inport
  Gain1 : Gain  Gain=0.017
  Gain2 : Gain  Gain=1/0.008
  Integrator1 : Integrator
  Sum4 : Sum  Inputs=+|+
  Out1 : Outport
  wires:
  Integrator1/1 -> Sum4/2
  Gain1/1 -> Gain2/1, Sum4/1
  Gain2/1 -> Integrator1/1
  Sum4/1 -> Out1/1
  In1/1 -> Gain1/1

== system simulation_version2021b/Aktor(Fadenzugmotor)3/PID_Regler_Pos. ==
  In1 : Inport
  Gain3 : Gain  Gain=4
  Out1 : Outport
  wires:
  Gain3/1 -> Out1/1
  In1/1 -> Gain3/1

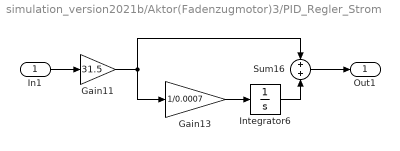
== system simulation_version2021b/Aktor(Fadenzugmotor)3/PID_Regler_Strom ==
  In1 : Inport
  Gain11 : Gain  Gain=31.5
  Gain13 : Gain  Gain=1/0.0007
  Integrator6 : Integrator
  Sum16 : Sum  Inputs=+|+
  Out1 : Outport
  wires:
  Gain13/1 -> Integrator6/1
  Gain11/1 -> Gain13/1, Sum16/1
  In1/1 -> Gain11/1
  Sum16/1 -> Out1/1
  Integrator6/1 -> Sum16/2

== system simulation_version2021b/Aktor(Servoverstäker+Fadenzugmotor)/Geschwindigkeitsvorsteuerung ==
  In1 : Inport
  Derivative : Derivative
  Gain : Gain
  Out1 : Outport
  wires:
  Derivative/1 -> Gain/1
  In1/1 -> Derivative/1
  Gain/1 -> Out1/1

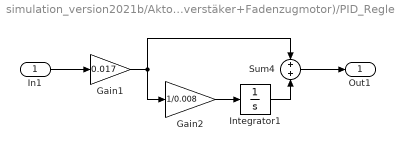
== system simulation_version2021b/Aktor(Servoverstäker+Fadenzugmotor)/PID_Regler_Ges. ==
  In1 : Inport
  Gain1 : Gain  Gain=0.017
  Gain2 : Gain  Gain=1/0.008
  Integrator1 : Integrator
  Sum4 : Sum  Inputs=+|+
  Out1 : Outport
  wires:
  Integrator1/1 -> Sum4/2
  Gain1/1 -> Gain2/1, Sum4/1
  Gain2/1 -> Integrator1/1
  Sum4/1 -> Out1/1
  In1/1 -> Gain1/1

== system simulation_version2021b/Aktor(Servoverstäker+Fadenzugmotor)/PID_Regler_Pos. ==
  In1 : Inport
  Gain3 : Gain  Gain=4
  Out1 : Outport
  wires:
  Gain3/1 -> Out1/1
  In1/1 -> Gain3/1

== system simulation_version2021b/Aktor(Servoverstäker+Fadenzugmotor)/PID_Regler_Strom ==
  In1 : Inport
  Gain11 : Gain  Gain=31.5
  Gain13 : Gain  Gain=1/0.0007
  Integrator6 : Integrator
  Sum16 : Sum  Inputs=+|+
  Out1 : Outport
  wires:
  Gain13/1 -> Integrator6/1
  Gain11/1 -> Gain13/1, Sum16/1
  In1/1 -> Gain11/1
  Sum16/1 -> Out1/1
  Integrator6/1 -> Sum16/2

== system simulation_version2021b/Aktor(Servoverstäker+Fadenzugmotor)1/Geschwindigkeitsvorsteuerung ==
  In1 : Inport
  Derivative : Derivative
  Gain : Gain
  Out1 : Outport
  wires:
  Derivative/1 -> Gain/1
  In1/1 -> Derivative/1
  Gain/1 -> Out1/1

== system simulation_version2021b/Aktor(Servoverstäker+Fadenzugmotor)1/PID_Regler_Ges. ==
  In1 : Inport
  Gain1 : Gain  Gain=0.017
  Gain2 : Gain  Gain=1/0.008
  Integrator1 : Integrator
  Sum4 : Sum  Inputs=+|+
  Out1 : Outport
  wires:
  Integrator1/1 -> Sum4/2
  Gain1/1 -> Gain2/1, Sum4/1
  Gain2/1 -> Integrator1/1
  Sum4/1 -> Out1/1
  In1/1 -> Gain1/1

== system simulation_version2021b/Aktor(Servoverstäker+Fadenzugmotor)1/PID_Regler_Pos. ==
  In1 : Inport
  Gain3 : Gain  Gain=4
  Out1 : Outport
  wires:
  Gain3/1 -> Out1/1
  In1/1 -> Gain3/1

== system simulation_version2021b/Aktor(Servoverstäker+Fadenzugmotor)1/PID_Regler_Strom ==
  In1 : Inport
  Gain11 : Gain  Gain=31.5
  Gain13 : Gain  Gain=1/0.0007
  Integrator6 : Integrator
  Sum16 : Sum  Inputs=+|+
  Out1 : Outport
  wires:
  Gain13/1 -> Integrator6/1
  Gain11/1 -> Gain13/1, Sum16/1
  In1/1 -> Gain11/1
  Sum16/1 -> Out1/1
  Integrator6/1 -> Sum16/2

== system simulation_version2021b/Aktor(Servoverstäker+Fadenzugmotor)2/Geschwindigkeitsvorsteuerung ==
  In1 : Inport
  Derivative : Derivative
  Gain : Gain
  Out1 : Outport
  wires:
  Derivative/1 -> Gain/1
  In1/1 -> Derivative/1
  Gain/1 -> Out1/1

== system simulation_version2021b/Aktor(Servoverstäker+Fadenzugmotor)2/PID_Regler_Ges. ==
  In1 : Inport
  Gain1 : Gain  Gain=0.017
  Gain2 : Gain  Gain=1/0.008
  Integrator1 : Integrator
  Sum4 : Sum  Inputs=+|+
  Out1 : Outport
  wires:
  Integrator1/1 -> Sum4/2
  Gain1/1 -> Gain2/1, Sum4/1
  Gain2/1 -> Integrator1/1
  Sum4/1 -> Out1/1
  In1/1 -> Gain1/1

== system simulation_version2021b/Aktor(Servoverstäker+Fadenzugmotor)2/PID_Regler_Pos. ==
  In1 : Inport
  Gain3 : Gain  Gain=4
  Out1 : Outport
  wires:
  Gain3/1 -> Out1/1
  In1/1 -> Gain3/1

== system simulation_version2021b/Aktor(Servoverstäker+Fadenzugmotor)2/PID_Regler_Strom ==
  In1 : Inport
  Gain11 : Gain  Gain=31.5
  Gain13 : Gain  Gain=1/0.0007
  Integrator6 : Integrator
  Sum16 : Sum  Inputs=+|+
  Out1 : Outport
  wires:
  Gain13/1 -> Integrator6/1
  Gain11/1 -> Gain13/1, Sum16/1
  In1/1 -> Gain11/1
  Sum16/1 -> Out1/1
  Integrator6/1 -> Sum16/2
